simulink model "realim_ref_dif0"  (R2019a)
settings: Solver=ode4  StartTime=0.0  StopTime=100  FixedStep=0.01  RelTol=1e-3
values from neighbouring files (symbols this model uses):
  K = Kaux(1:3)    [Control.m]
  L = Kaux(4)    [Control.m]
  operPoint = [x0(i); y0(i); z0(i)]    [Control.m]
  systemD = c2d(system,1)    [Control.m]
  T = 1    [Control.m]
settings Model: Creator=Mateo  LastModifiedBy=Juan
settings DataIOCC: SaveFormat=Array  SignalLogging=off  DSMLogging=off  ReturnWorkspaceOutputs=off

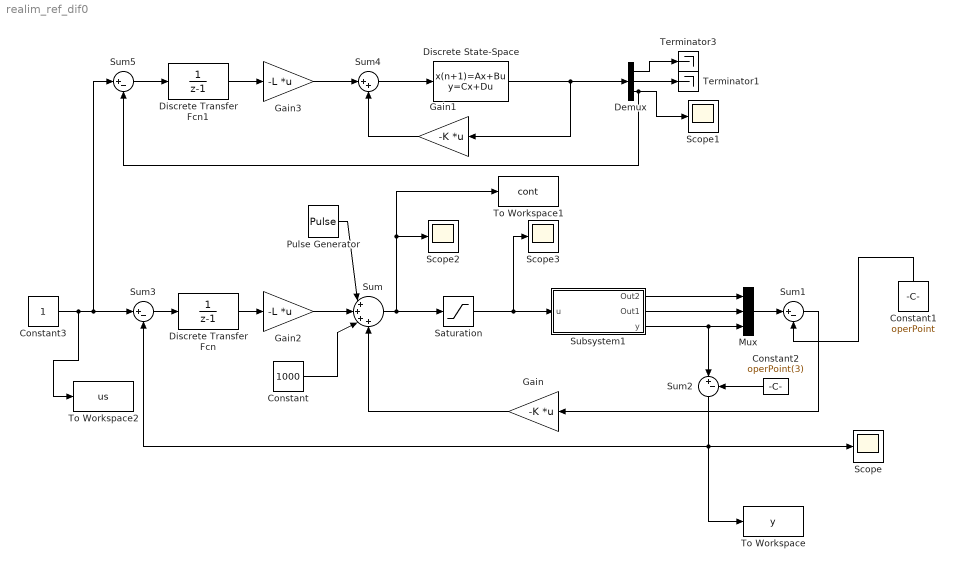
== system realim_ref_dif0 ==
  Constant : Constant  Value=1000
  Constant1 : Constant  Value=operPoint
  Constant2 : Constant  Value=operPoint(3)
  Constant3 : Constant
  Demux : Demux  Outputs=3
  Discrete Transfer Fcn : DiscreteTransferFcn  Denominator=[1 -1]  SampleTime=T
  Discrete Transfer Fcn1 : DiscreteTransferFcn  Denominator=[1 -1]  SampleTime=T
  Discrete State-Space : DiscreteStateSpace  A=systemD.A  B=systemD.B  C=eye(3)  D=[0,0,0]'  InitialCondition=[0,0,0]
  Gain : Gain  Gain=-K  Multiplication=Matrix(K*u) (u vector)
  Gain1 : Gain  Gain=-K  Multiplication=Matrix(K*u) (u vector)
  Gain2 : Gain  Gain=-L  Multiplication=Matrix(K*u) (u vector)
  Gain3 : Gain  Gain=-L  Multiplication=Matrix(K*u) (u vector)
  Mux : Mux  Inputs=3
  Pulse Generator : DiscretePulseGenerator  PulseType=Time based  Amplitude=0  Period=10  PulseWidth=5
  Saturation : Saturate  UpperLimit=1500  LowerLimit=0
  Scope{,1..3} (4 alike) : Scope
  Subsystem1 : Subsystem  mask{Ra=250, Rb=7500, Rc=17.5439, RCs=1, ci=[0.522807167562789;-2.614035837813944;2.614035837813944]}
      mask prompts: Ra "Resistance a"; Rb "Resistance b"; Rc "Resistance c"; RCs "Time speed (RC)"; ci "Initial Conditions"
      mask init:
      | x10 = ci(1);
      | x20 = ci(2);
      | y0 = ci(3);
      mask Display: disp("Rössler Attractor")
  Sum : Sum  Inputs=|++++
  Sum{1..3,5} (4 alike) : Sum  Inputs=|+-
  Sum4 : Sum  Inputs=|++
  Terminator1 : Terminator
  Terminator3 : Terminator
  To Workspace : ToWorkspace  VariableName=y  SampleTime=-1
  To Workspace1 : ToWorkspace  VariableName=cont  SampleTime=-1
  To Workspace2 : ToWorkspace  VariableName=us  SampleTime=-1
  wires:
  Saturation/1 -> Subsystem1/1(u), Scope3/1
  Discrete State-Space/1 -> Gain1/1, Demux/1
  Mux/1 -> Sum1/1
  Subsystem1/1(Out2) -> Mux/1
  Subsystem1/3("y ") -> Mux/3, Sum2/1
  Constant1/1 -> Sum1/2
  Demux/1 -> Terminator3/1
  Demux/3 -> Sum5/2, Scope1/1
  Sum2/1 -> To Workspace/1, Scope/1, Sum3/2
  Demux/2 -> Terminator1/1
  Constant2/1 -> Sum2/2
  Subsystem1/2(Out1) -> Mux/2
  Sum/1 -> Saturation/1, To Workspace1/1, Scope2/1
  Sum1/1 -> Gain/1
  Constant3/1 -> To Workspace2/1, Sum3/1, Sum5/1
  Sum3/1 -> Discrete Transfer Fcn/1
  Discrete Transfer Fcn/1 -> Gain2/1
  Gain/1 -> Sum/4
  Sum4/1 -> Discrete State-Space/1
  Gain1/1 -> Sum4/2
  Gain3/1 -> Sum4/1
  Discrete Transfer Fcn1/1 -> Gain3/1
  Sum5/1 -> Discrete Transfer Fcn1/1
  Constant/1 -> Sum/3
  Gain2/1 -> Sum/2
  Pulse Generator/1 -> Sum/1

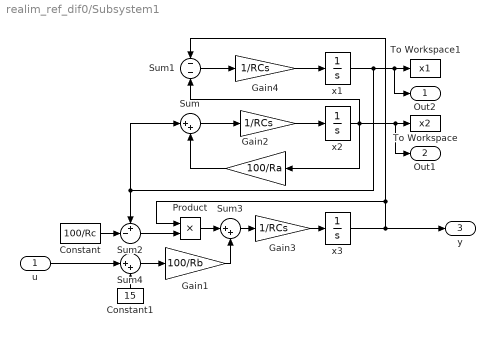
== system realim_ref_dif0/Subsystem1 ==
  u : Inport
  " " : Gain  Gain=1/RCs
  Constant : Constant  Value=100/Rc
  Constant1 : Constant  Value=15
  Gain1 : Gain  Gain=100/Rb
  Gain2 : Gain  Gain=100/Ra
  Gain3 : Gain  Gain=1/RCs
  Gain4 : Gain  Gain=1/RCs
  Product : Product
  Sum : Sum  Inputs=|++
  Sum1 : Sum  Inputs=--
  Sum2 : Sum  Inputs=+-|
  Sum3 : Sum  Inputs=|++
  Sum4 : Sum  Inputs=|++
  To Workspace : ToWorkspace  VariableName=x2  SampleTime=-1
  To Workspace1 : ToWorkspace  VariableName=x1  SampleTime=-1
  x1 : Integrator  InitialCondition=x10
  x2 : Integrator  InitialCondition=x20
  "x3 " : Integrator  InitialCondition=y0
  Out2 : Outport
  Out1 : Outport  Port=2
  "y " : Outport  Port=3
  wires:
  Sum4/1 -> Gain1/1
  Constant1/1 -> Sum4/2
  Gain1/1 -> Sum3/2
  Gain4/1 -> x1/1
  Gain3/1 -> "x3 "/1
  " "/1 -> x2/1
  u/1 -> Sum4/1
  x2/1 -> Gain2/1, To Workspace/1, Out1/1, Sum1/2
  Constant/1 -> Sum2/2
  Sum3/1 -> Gain3/1
  Sum/1 -> " "/1
  x1/1 -> Sum/1, Sum2/1, To Workspace1/1, Out2/1
  "x3 "/1 -> Product/1, Sum1/1, "y "/1
  Product/1 -> Sum3/1
  Sum2/1 -> Product/2
  Gain2/1 -> Sum/2
  Sum1/1 -> Gain4/1
